simulink model "motordriver"  (R2015b)
settings: Solver=ode4  StartTime=0.0  StopTime=10  FixedStep=0.0002  RelTol=1e-3
undefined symbols (not defined in the file or in its folder): alpha, Ki, Kp, tau
settings Model: ExtModeTrigDuration=10000  Creator=millerid  LastModifiedBy=millerid
settings SolverCC: PositivePriorityOrder=on
settings RTWCC: SystemTargetFile=quarc_win64.tlc  TemplateMakefile=quarc_default_tmf  Description=QUARC Win64 Target
settings STFCustomTargetCC: TargetPreCompLibLocation=C:\ProgramData\QUARC\lib\2015b\win64\release  GeneratePreprocessorConditionals=Use local settings  CPPClassGenCompliant=off
settings GRTTargetCC: TargetPreCompLibLocation=C:\ProgramData\QUARC\lib\2015b\win64\release  ParMdlRefBuildCompliant=off  CompOptLevelCompliant=off  CombineOutputUpdateFcns=off  MatFileLogging=off  CPPClassGenCompliant=off  GRTInterface=on  UseToolchainInfoCompliant=off  ExtMode=on  ExtModeMexFile=quarc_comm

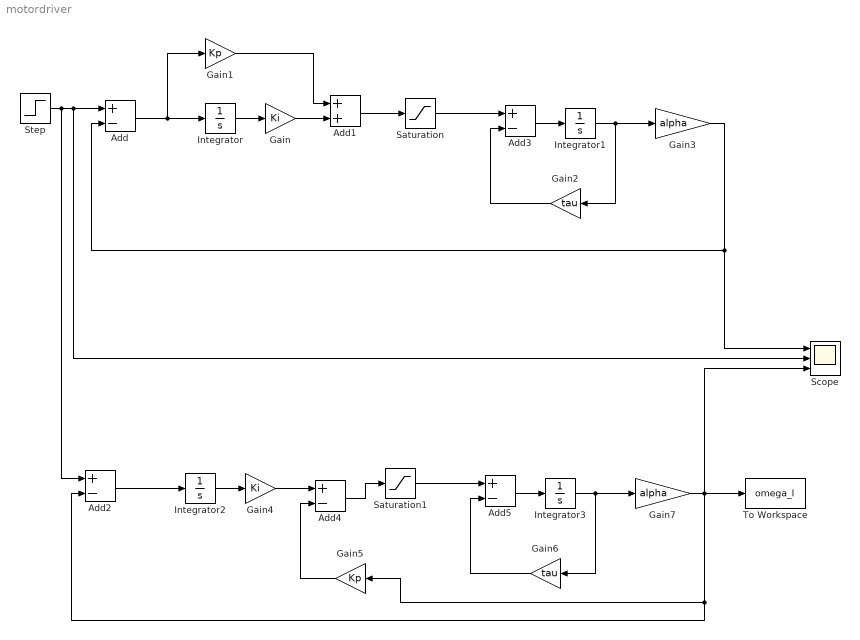
== system motordriver ==
  Add{,2..5} (5 alike) : Sum  Inputs=+-
  Add1 : Sum
  Gain : Gain  Gain=Ki
  Gain1 : Gain  Gain=Kp
  Gain2 : Gain  Gain=tau
  Gain3 : Gain  Gain=alpha
  Gain4 : Gain  Gain=Ki
  Gain5 : Gain  Gain=Kp
  Gain6 : Gain  Gain=tau
  Gain7 : Gain  Gain=alpha
  Integrator{,1..3} (4 alike) : Integrator
  Saturation : Saturate  UpperLimit=10  LowerLimit=-10
  Saturation1 : Saturate  UpperLimit=10  LowerLimit=-10
  Scope : Scope  NumInputPorts=3
  Step : Step  Time=0  After=7.5  SampleTime=0
  To Workspace : ToWorkspace  VariableName=omega_l  SaveFormat=Timeseries  SampleTime=-1
  wires:
  Add/1 -> Gain1/1, Integrator/1
  Integrator/1 -> Gain/1
  Gain/1 -> Add1/2
  Gain1/1 -> Add1/1
  Add1/1 -> Saturation/1
  Integrator1/1 -> Gain3/1, Gain2/1
  Gain2/1 -> Add3/2
  Add3/1 -> Integrator1/1
  Saturation/1 -> Add3/1
  Gain3/1 -> Scope/1, Add/2
  Add2/1 -> Integrator2/1
  Integrator2/1 -> Gain4/1
  Gain4/1 -> Add4/1
  Add4/1 -> Saturation1/1
  Integrator3/1 -> Gain7/1, Gain6/1
  Gain6/1 -> Add5/2
  Add5/1 -> Integrator3/1
  Saturation1/1 -> Add5/1
  Gain7/1 -> Scope/3, To Workspace/1, Gain5/1, Add2/2
  Step/1 -> Add2/1, Scope/2, Add/1
  Gain5/1 -> Add4/2
